simulink model "DISCON_FFFB_IEA15MW"  (R2024a)
settings: Solver=FixedStepDiscrete  StartTime=0.0  StopTime=inf  FixedStep=Ts  RelTol=1e-3
settings Model: Creator=evansolingen  LastModifiedBy=glazzerini
settings SolverCC: AlgebraicLoopSolver=TrustRegion
settings DataIOCC: LimitDataPoints=on  SaveFormat=Array  SignalLoggingSaveFormat=ModelDataLogs  SaveOutput=off  SignalLogging=off  SaveTime=off  ReturnWorkspaceOutputs=off
settings OptimizationCC: ExpressionDepthLimit=2147483647  LifeSpan=inf
settings DebuggingCC: UnderspecifiedInitializationDetection=Classic  MergeDetectMultiDrivingBlocksExec=none  SolverPrmCheckMsg=warning  MultiTaskDSMMsg=warning  MultiTaskCondExecSysMsg=none  FcnCallInpInsideContextMsg=warning  UnconnectedInputMsg=warning  UnconnectedOutputMsg=warning  UnconnectedLineMsg=warning  AllowSymbolicDim=off  StateNameClashWarn=warning  SFUnexpectedBacktrackingDiag=warning  SFNoUnconditionalDefaultTransitionDiag=warning  SFExecutionAtInitializationDiag=none  ArithmeticOperatorsInVariantConditions=warning
settings HardwareCC: ProdBitPerPointer=32  ProdBitPerSizeT=32  ProdBitPerPtrDiffT=32  ProdLargestAtomicFloat=None  ProdIntDivRoundTo=Undefined  ProdEndianess=Unspecified  ProdWordSize=32  ProdHWDeviceType=32-bit Generic
settings ModelReferenceCC: UpdateModelReferenceTargets=Force  EnableRefExpFcnMdlSchedulingChecks=on  PropagateSignalLabelsOutOfModel=off
settings SFSimCC: SimUseLocalCustomCode=off  SimParseCustomCode=off  CustomCodeUndefinedFunction=UseInterfaceOnly
settings RTWCC: Description=DISCON DLL Target (for use with GH BLADED)  SystemTargetFile=discon.tlc  TemplateMakefile=discon_vc.tmf  RTWUseLocalCustomCode=off  GPUComputeCapability=3.5  DLArmComputeVersion=19.05
settings CodeAppCC: StateflowObjectComments=on
settings GRTTargetCC: TargetLangStandard=C89/C90 (ANSI)  CombineOutputUpdateFcns=off  GRTInterface=on  UseToolchainInfoCompliant=off  ExtModeMexFile=noextcomm
settings ConfigComp: CovMetricSettings=dw  CovSaveCumulativeToWorkspaceVar=on  CovSaveSingleToWorkspaceVar=on  CovExternalEMLEnable=off

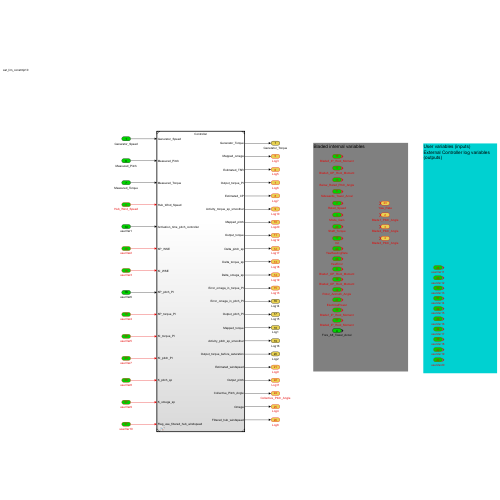
[thumbnail: Simulink's stored preview of the top-level diagram]
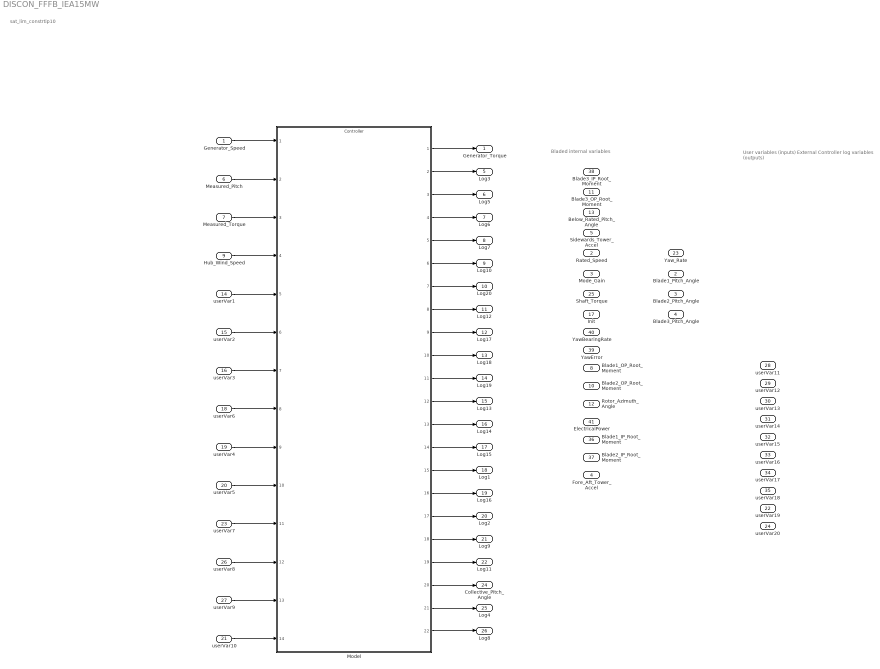
== system DISCON_FFFB_IEA15MW ==
  note: sat_lim_constrtip10
  note: Bladed internal variables
  note: User variables (inputs)
      | External Controller log variables (outputs)
  Generator_Speed : Inport
  Rated_Speed : Inport  Port=2  PortDimensions=1
  Mode_Gain : Inport  Port=3  PortDimensions=1
  Fore_Aft_Tower_Accel : Inport  Port=4  PortDimensions=1
  Sidewards_Tower_Accel : Inport  Port=5  PortDimensions=1
  Measured_Pitch : Inport  Port=6  PortDimensions=1
  Measured_Torque : Inport  Port=7  PortDimensions=1
  Blade1_OP_Root_Moment : Inport  Port=8  PortDimensions=1
  Hub_Wind_Speed : Inport  Port=9  PortDimensions=1
  Blade2_OP_Root_Moment : Inport  Port=10  PortDimensions=1
  Blade3_OP_Root_Moment : Inport  Port=11  PortDimensions=1
  Rotor_Azimuth_Angle : Inport  Port=12  PortDimensions=1
  Below_Rated_Pitch_Angle : Inport  Port=13  PortDimensions=1
  userVar1 : Inport  Port=14  PortDimensions=1
  userVar2 : Inport  Port=15  PortDimensions=1
  userVar3 : Inport  Port=16  PortDimensions=1
  Init : Inport  Port=17  PortDimensions=1
  userVar6 : Inport  Port=18  PortDimensions=1
  userVar4 : Inport  Port=19  PortDimensions=1
  userVar5 : Inport  Port=20  PortDimensions=1
  userVar10 : Inport  Port=21  PortDimensions=1
  userVar19 : Inport  Port=22  PortDimensions=1
  userVar7 : Inport  Port=23  PortDimensions=1
  userVar20 : Inport  Port=24  PortDimensions=1
  Shaft_Torque : Inport  Port=25  PortDimensions=1
  userVar8 : Inport  Port=26  PortDimensions=1
  userVar9 : Inport  Port=27  PortDimensions=1
  userVar11 : Inport  Port=28  PortDimensions=1
  userVar12 : Inport  Port=29  PortDimensions=1
  userVar13 : Inport  Port=30  PortDimensions=1
  userVar14 : Inport  Port=31  PortDimensions=1
  userVar15 : Inport  Port=32  PortDimensions=1
  userVar16 : Inport  Port=33  PortDimensions=1
  userVar17 : Inport  Port=34  PortDimensions=1
  userVar18 : Inport  Port=35  PortDimensions=1
  Blade1_IP_Root_Moment : Inport  Port=36  PortDimensions=1
  Blade2_IP_Root_Moment : Inport  Port=37  PortDimensions=1
  Blade3_IP_Root_Moment : Inport  Port=38  PortDimensions=1
  YawError : Inport  Port=39  PortDimensions=1
  YawBearingRate : Inport  Port=40  PortDimensions=1
  ElectricalPower : Inport  Port=41  PortDimensions=1
  Model : ModelReference  ModelNameDialog=Controller.slx  SimulationMode=Normal  ModelReferenceVersion=18.123
  Generator_Torque : Outport
  Blade1_Pitch_Angle : Outport  Port=2  PortDimensions=1
  Blade2_Pitch_Angle : Outport  Port=3  PortDimensions=1
  Blade3_Pitch_Angle : Outport  Port=4  PortDimensions=1
  Log3 : Outport  Port=5  PortDimensions=1
  Log5 : Outport  Port=6  PortDimensions=1
  Log6 : Outport  Port=7  PortDimensions=1
  Log7 : Outport  Port=8  PortDimensions=1
  Log10 : Outport  Port=9  PortDimensions=1
  Log20 : Outport  Port=10  PortDimensions=1
  Log12 : Outport  Port=11  PortDimensions=1
  Log17 : Outport  Port=12  PortDimensions=1
  Log18 : Outport  Port=13  PortDimensions=1
  Log19 : Outport  Port=14  PortDimensions=1
  Log13 : Outport  Port=15  PortDimensions=1
  Log14 : Outport  Port=16  PortDimensions=1
  Log15 : Outport  Port=17  PortDimensions=1
  Log1 : Outport  Port=18  PortDimensions=1
  Log16 : Outport  Port=19  PortDimensions=1
  Log2 : Outport  Port=20  PortDimensions=1
  Log9 : Outport  Port=21  PortDimensions=1
  Log11 : Outport  Port=22  PortDimensions=1
  Yaw_Rate : Outport  Port=23  PortDimensions=1
  Collective_Pitch_Angle : Outport  Port=24  PortDimensions=1
  Log4 : Outport  Port=25  PortDimensions=1
  Log8 : Outport  Port=26  PortDimensions=1
  wires:
  userVar1/1 -> Model/5
  Model/20 -> Collective_Pitch_Angle/1
  userVar6/1 -> Model/8
  Model/18 -> Log9/1
  Model/7 -> Log20/1
  Model/6 -> Log10/1
  userVar2/1 -> Model/6
  userVar3/1 -> Model/7
  Model/8 -> Log12/1
  Model/3 -> Log5/1
  Model/14 -> Log15/1
  Model/1 -> Generator_Torque/1
  Model/2 -> Log3/1
  Model/17 -> Log2/1
  Model/11 -> Log19/1
  Model/12 -> Log13/1
  Model/13 -> Log14/1
  Model/4 -> Log6/1
  Model/9 -> Log17/1
  Model/16 -> Log16/1
  Model/15 -> Log1/1
  Model/10 -> Log18/1
  Model/5 -> Log7/1
  Model/19 -> Log11/1
  Model/21 -> Log4/1
  Model/22 -> Log8/1
  Measured_Pitch/1 -> Model/2
  Generator_Speed/1 -> Model/1
  Measured_Torque/1 -> Model/3
  Hub_Wind_Speed/1 -> Model/4
  userVar7/1 -> Model/11
  userVar4/1 -> Model/9
  userVar5/1 -> Model/10
  userVar9/1 -> Model/13
  userVar8/1 -> Model/12
  userVar10/1 -> Model/14
